simulink model "beeper"  (R2018b)
settings: Solver=ode3  StartTime=0.0  StopTime=10  RelTol=1e-3  EnableMultiTasking=on
libraries: legoev3lib x3
settings Model: FPTRunName=Active  ExtModeTrigDuration=2  Creator=Sjoerd  LastModifiedBy=Sjoerd
settings SolverCC: PositivePriorityOrder=on
settings DataIOCC: LimitDataPoints=on  SaveFormat=Array
settings OptimizationCC: ExpressionDepthLimit=2147483647  LifeSpan=Inf  MaxStackSize=64
settings DebuggingCC: UnderspecifiedInitializationDetection=Classic  MergeDetectMultiDrivingBlocksExec=none  FcnCallInpInsideContextMsg=warning  AllowSymbolicDim=off  StateNameClashWarn=warning  SFUnexpectedBacktrackingDiag=warning  SFNoUnconditionalDefaultTransitionDiag=warning  SFExecutionAtInitializationDiag=none
settings HardwareCC: ProdBitPerPointer=32  ProdBitPerSizeT=32  ProdBitPerPtrDiffT=32  ProdLargestAtomicInteger=Long  ProdWordSize=32  ProdHWDeviceType=ARM Compatible->ARM 9  UseEmbeddedCoderFeatures=off  UseSimulinkCoderFeatures=off
settings ModelReferenceCC: PropagateSignalLabelsOutOfModel=off
settings SFSimCC: SimUseLocalCustomCode=off
settings RTWCC: SystemTargetFile=ert.tlc  HardwareBoard=LEGO MINDSTORMS EV3  TemplateMakefile=ert_default_tmf  GenerateReport=on  RTWVerbose=off  RTWUseLocalCustomCode=off  Toolchain=Sourcery G++ Lite v2009q3  BuildConfiguration=Faster Runs  LaunchReport=on
settings CodeAppCC: ForceParamTrailComments=on  OperatorAnnotations=on  StateflowObjectComments=on  MATLABSourceComments=on
settings ERTTargetCC: MultiwordLength=2048  ERTCustomFileBanners=off  SupportContinuousTime=on  SupportNonInlinedSFcns=on  RemoveResetFunc=off  SupportVariableSizeSignals=on  ModelStepFunctionPrototypeControlCompliant=off
settings ConfigComp: CovMetricSettings=dw  CovHtmlReporting=on  CovSaveCumulativeToWorkspaceVar=on  CovSaveSingleToWorkspaceVar=on  CovExternalEMLEnable=off  CovSFcnEnable=off

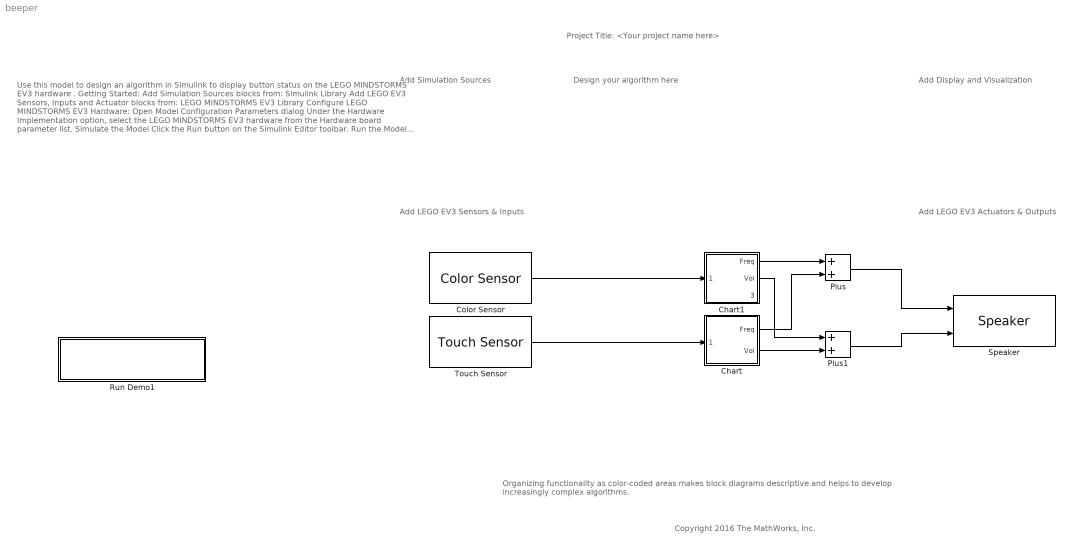
== system beeper ==
  note: Project Title: <Your project name here>
  note: Copyright 2016 The MathWorks, Inc.
  note: Add LEGO EV3 Sensors & Inputs
  note: Add LEGO EV3 Actuators & Outputs
  note: Add Display and Visualization
  note: Design your algorithm here
  note: Add Simulation Sources
  note: Use this model to design an algorithm in Simulink to display button status on the LEGO MINDSTORMS EV3 hardware .
      |
      | Getting Started:
      |
      | Add Simulation Sources blocks from:
      | Simulink Library
      | Add LEGO EV3 Sensors, Inputs and Actuator blocks from:
      | LEGO MINDSTORMS EV3 Library
      |
      | Configure LEGO MINDSTORMS EV3 Hardware:
      |
      | Open Model Configuration Parameters dialog
      | Under the Hardware Implementation option, select the LEGO MINDSTORMS EV3 hardware from the Hardware board parameter list.
      |
      | Simulate the Model
      |
      | Click the Run button on the Simulink Editor toolbar.
      |
      | Run the Model on LEGO MINDSTORMS EV3 Hardware
      |
      | Click the Deploy to Hardware button on the Simulink Editor toolbar.
      |
      | Other Things to Try:
      |
      | Create and run a model that detects the obstacle and stops the LEGO EV3 robot. HINT: Use Ultrasonic Sensor and Motor blocks.
  note: Organizing functionality as color-coded areas makes block diagrams descriptive and helps to develop increasingly complex algorithms.
  Chart : Stateflow chart  TreatAsAtomicUnit=on
  Chart1 : Stateflow chart  TreatAsAtomicUnit=on
  Color Sensor : legoev3lib/Color Sensor  portNumber=3  mode=Color  sampleTime=0.1
      settings: SourceProductName=Simulink Support Package for LEGO MINDSTORMS EV3 Hardware  SourceProductBaseCode=LEGOEV3
  Plus : Sum
  Plus1 : Sum
  Run Demo1 : Subsystem  Description=Controls host-side RTDX processing.
      mask Display: pic=imread('ev3DeploytoHardware.png');image(pic);
  Speaker : legoev3lib/Speaker  sinputMode=Frequency and volume  sspeakerFreq=32  sspeakerVolume=50  sspeakerDuration=500
      settings: SourceProductName=Simulink Support Package for LEGO MINDSTORMS EV3 Hardware  SourceProductBaseCode=LEGOEV3
  Touch Sensor : legoev3lib/Touch Sensor  portNumber=1  sampleTime=0.1
      settings: SourceProductName=Simulink Support Package for LEGO MINDSTORMS EV3 Hardware  SourceProductBaseCode=LEGOEV3
  wires:
  Touch Sensor/1 -> Chart/1(button)
  Chart/1(Freq) -> Plus/2
  Color Sensor/1 -> Chart1/1(button)
  Chart1/1(Freq) -> Plus/1
  Plus/1 -> Speaker/1
  Plus1/1 -> Speaker/2
  Chart/2(Vol) -> Plus1/2
  Chart1/2(Vol) -> Plus1/1

== system beeper/Run Demo1 ==

== stateflow chart beeper/Chart1 ==
  state a
  state b
    Vol = 20
    Freq = 32
  state c
    Vol = 0
    Freq = 0
  (default) -> a : {Vol = 0;
      | Freq = 0}
  a -> b : [button == 1]{myevent}
  c -> a
  b -> c : [button ~= 1]
  data: button input; Freq output; Vol output
  events: myevent output FUNCTION_CALL_EVENT

== stateflow chart beeper/Chart ==
  state a
  state b
    Vol = 20
    Freq = 64
  state c
    Vol = 0
    Freq = 0
  (default) -> a : {Vol = 0;
      | Freq = 0}
  a -> b : [button == 1]
  c -> a
  b -> c : [button == 0]
  data: button input; Freq output; Vol output
